simulink model "lab_3_task_3_simulink"  (R2025b)
settings: Solver=ode5  StartTime=0.0  StopTime=16  FixedStep=0.01  RelTol=1e-3
values from neighbouring files (symbols this model uses):
  ix = 0.070    (= 0.07)    [lab_3_task_1.m]    (also in lab_3_task_2.m = 0.0504; lab_3_task_3.m = 0.025; lab_3_task_4.m; lab_4_task_1.m)
  iy = 0.055    [lab_3_task_1.m]    (also in lab_3_task_2.m = 0.0504; lab_3_task_3.m; lab_3_task_4.m = 0.0109; lab_4_task_1.m)
  iz = 0.025    [lab_3_task_1.m]    (also in lab_3_task_2.m = 0.0109; lab_3_task_3.m = 0.07; lab_3_task_4.m = 0.0504; lab_4_task_1.m)
  wx0 = 0.45    [lab_3_task_1.m]    (also in lab_3_task_2.m = 0.1; lab_3_task_3.m = w0(1); lab_3_task_4.m = 1e-06; lab_4_task_1.m)
  wy0 = 0.52    [lab_3_task_1.m]    (also in lab_3_task_2.m = 0.1; lab_3_task_3.m = w0(2); lab_3_task_4.m = 1e-06; lab_4_task_1.m)
  wz0 = 0.55    [lab_3_task_1.m]    (also in lab_3_task_2.m = 0.1; lab_3_task_3.m = w0(3); lab_3_task_4.m = 0.02; lab_4_task_1.m)
settings Model: Creator=User  LastModifiedBy=User

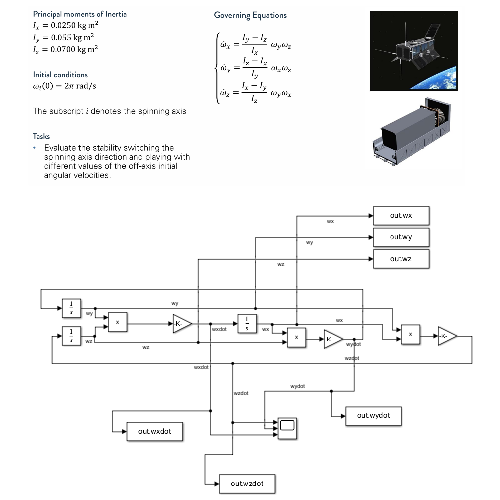
[thumbnail: Simulink's stored preview of the top-level diagram]
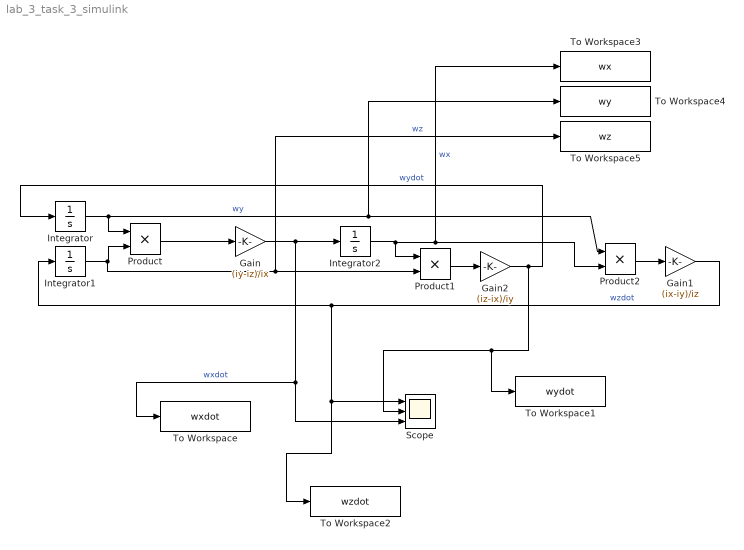
== system lab_3_task_3_simulink ==
  Gain : Gain  Gain=(iy-iz)/ix
  Gain1 : Gain  Gain=(ix-iy)/iz
  Gain2 : Gain  Gain=(iz-ix)/iy
  Integrator : Integrator  InitialCondition=wy0
  Integrator1 : Integrator  InitialCondition=wz0
  Integrator2 : Integrator  InitialCondition=wx0
  Product : Product
  Product1 : Product
  Product2 : Product
  Scope : Scope  NumInputPorts=3
      settings: ActiveDisplayYMinimum=-0.42457603967865376  ActiveDisplayYMaximum=0.42457603981533126
  To Workspace : ToWorkspace  VariableName=wxdot  SaveFormat=Timeseries  SampleTime=-1
  To Workspace1 : ToWorkspace  VariableName=wydot  SaveFormat=Timeseries  SampleTime=-1
  To Workspace2 : ToWorkspace  VariableName=wzdot  SaveFormat=Timeseries  SampleTime=-1
  To Workspace3 : ToWorkspace  VariableName=wx  SaveFormat=Timeseries  SampleTime=-1
  To Workspace4 : ToWorkspace  VariableName=wy  SaveFormat=Timeseries  SampleTime=-1
  To Workspace5 : ToWorkspace  VariableName=wz  SaveFormat=Timeseries  SampleTime=-1
  wires:
  Integrator2/1 -> To Workspace3/1, Product2/2, Product1/1  "wx"
  Product1/1 -> Gain2/1
  Product2/1 -> Gain1/1
  Gain2/1 -> To Workspace1/1, Scope/2, Integrator/1  "wydot"
  Gain1/1 -> To Workspace2/1, Scope/1, Integrator1/1  "wzdot"
  Product/1 -> Gain/1
  Integrator1/1 -> To Workspace5/1, Product1/2, Product/2  "wz"
  Integrator/1 -> To Workspace4/1, Product2/1, Product/1  "wy"
  Gain/1 -> To Workspace/1, Scope/3, Integrator2/1  "wxdot"
